simulink model "c2837xD_lcd_display"  (R2021b)
settings: Solver=FixedStepDiscrete  StartTime=0.0  StopTime=Inf  RelTol=1e-3  EnableMultiTasking=on
InitFcn:
  | c2837xD_Display_Param;
values from neighbouring files (symbols this model uses):
  SCI_counter = SCI_ping_buffer_size/SCI_chunk_size    (= 640)    [c2837xD_Display_Param.m]
  SCI_ping_buffer_size = image_height*lines_in_packet    (= 3840)    [c2837xD_Display_Param.m]
  TI_chunk_size = SCI_chunk_size    (= 6)    [c2837xD_Display_Param.m]
  TI_ping_buffer_size = SCI_ping_buffer_size    (= 3840)    [c2837xD_Display_Param.m]
libraries: c280xlib x63, c2837xDlib x63, simulink x41, c2000lib x1, demo_controls x1, dspswit3 x1, idelinklib_common x1
(part 2 of 4)

== system c2837xD_lcd_display/Initialization/GammaCorrection1/Subsystem1 ==
  Cmd : Inport
  Data : Inport  Port=2
  function : TriggerPort  TriggerType=function-call  VariantControl=Variant
  Function-Call Generator : simulink/Ports & Subsystems/Function-Call Generator  sample_time=-1  numberOfIterations=1  DisallowWideOutput=off
  Function-Call Split : FunctionCallSplit  NumOutputPorts=2
  Function-Call Split1 : FunctionCallSplit  NumOutputPorts=2
  Function-Call Split4 : FunctionCallSplit  NumOutputPorts=2
  SendCommand : Subsystem
  SendData : Subsystem
  SetCmd : Subsystem  TreatAsAtomicUnit=on
  SetData : Subsystem  TreatAsAtomicUnit=on
  wires:
  Function-Call Split1/2 -> Function-Call Split4/1
  Function-Call Split/2 -> Function-Call Split1/1
  Data/1 -> SendData/1(Data)
  Function-Call Generator/1 -> Function-Call Split/1
  Function-Call Split/1 -> SetCmd/Trigger
  Function-Call Split4/2 -> SendData/Trigger
  Function-Call Split4/1 -> SetData/Trigger
  Function-Call Split1/1 -> SendCommand/Trigger
  Cmd/1 -> SendCommand/1(cmd)

== system c2837xD_lcd_display/Initialization/GammaCorrection1/Subsystem2 ==
  Cmd : Inport
  Data : Inport  Port=2
  function : TriggerPort  TriggerType=function-call  VariantControl=Variant
  Function-Call Generator : simulink/Ports & Subsystems/Function-Call Generator  sample_time=-1  numberOfIterations=1  DisallowWideOutput=off
  Function-Call Split : FunctionCallSplit  NumOutputPorts=2
  Function-Call Split1 : FunctionCallSplit  NumOutputPorts=2
  Function-Call Split4 : FunctionCallSplit  NumOutputPorts=2
  SendCommand : Subsystem
  SendData : Subsystem
  SetCmd : Subsystem  TreatAsAtomicUnit=on
  SetData : Subsystem  TreatAsAtomicUnit=on
  wires:
  Function-Call Split1/2 -> Function-Call Split4/1
  Function-Call Split/2 -> Function-Call Split1/1
  Data/1 -> SendData/1(Data)
  Function-Call Generator/1 -> Function-Call Split/1
  Function-Call Split/1 -> SetCmd/Trigger
  Function-Call Split4/2 -> SendData/Trigger
  Function-Call Split4/1 -> SetData/Trigger
  Function-Call Split1/1 -> SendCommand/Trigger
  Cmd/1 -> SendCommand/1(cmd)

== system c2837xD_lcd_display/Initialization/GammaCorrection1/Subsystem3 ==
  Cmd : Inport
  Data : Inport  Port=2
  function : TriggerPort  TriggerType=function-call  VariantControl=Variant
  Function-Call Generator : simulink/Ports & Subsystems/Function-Call Generator  sample_time=-1  numberOfIterations=1  DisallowWideOutput=off
  Function-Call Split : FunctionCallSplit  NumOutputPorts=2
  Function-Call Split1 : FunctionCallSplit  NumOutputPorts=2
  Function-Call Split4 : FunctionCallSplit  NumOutputPorts=2
  SendCommand : Subsystem
  SendData : Subsystem
  SetCmd : Subsystem  TreatAsAtomicUnit=on
  SetData : Subsystem  TreatAsAtomicUnit=on
  wires:
  Function-Call Split1/2 -> Function-Call Split4/1
  Function-Call Split/2 -> Function-Call Split1/1
  Data/1 -> SendData/1(Data)
  Function-Call Generator/1 -> Function-Call Split/1
  Function-Call Split/1 -> SetCmd/Trigger
  Function-Call Split4/2 -> SendData/Trigger
  Function-Call Split4/1 -> SetData/Trigger
  Function-Call Split1/1 -> SendCommand/Trigger
  Cmd/1 -> SendCommand/1(cmd)

== system c2837xD_lcd_display/Initialization/GammaCorrection1/Subsystem4 ==
  Cmd : Inport
  Data : Inport  Port=2
  function : TriggerPort  TriggerType=function-call  VariantControl=Variant
  Function-Call Generator : simulink/Ports & Subsystems/Function-Call Generator  sample_time=-1  numberOfIterations=1  DisallowWideOutput=off
  Function-Call Split : FunctionCallSplit  NumOutputPorts=2
  Function-Call Split1 : FunctionCallSplit  NumOutputPorts=2
  Function-Call Split4 : FunctionCallSplit  NumOutputPorts=2
  SendCommand : Subsystem
  SendData : Subsystem
  SetCmd : Subsystem  TreatAsAtomicUnit=on
  SetData : Subsystem  TreatAsAtomicUnit=on
  wires:
  Function-Call Split1/2 -> Function-Call Split4/1
  Function-Call Split/2 -> Function-Call Split1/1
  Data/1 -> SendData/1(Data)
  Function-Call Generator/1 -> Function-Call Split/1
  Function-Call Split/1 -> SetCmd/Trigger
  Function-Call Split4/2 -> SendData/Trigger
  Function-Call Split4/1 -> SetData/Trigger
  Function-Call Split1/1 -> SendCommand/Trigger
  Cmd/1 -> SendCommand/1(cmd)

== system c2837xD_lcd_display/Initialization/InitPwr/Subsystem ==
  Cmd : Inport
  Data : Inport  Port=2
  Function-Call Generator : simulink/Ports & Subsystems/Function-Call Generator  sample_time=-1  numberOfIterations=1  DisallowWideOutput=off
  Function-Call Split : FunctionCallSplit  NumOutputPorts=2
  Function-Call Split1 : FunctionCallSplit  NumOutputPorts=2
  Function-Call Split4 : FunctionCallSplit  NumOutputPorts=2
  SendCommand : Subsystem
  SendData : Subsystem
  SetCmd : Subsystem  TreatAsAtomicUnit=on
  SetData : Subsystem  TreatAsAtomicUnit=on
  wires:
  Function-Call Split1/1 -> SendCommand/Trigger
  Function-Call Generator/1 -> Function-Call Split/1
  Function-Call Split/1 -> SetCmd/Trigger
  Function-Call Split4/2 -> SendData/Trigger
  Function-Call Split4/1 -> SetData/Trigger
  Data/1 -> SendData/1(Data)
  Cmd/1 -> SendCommand/1(cmd)
  Function-Call Split1/2 -> Function-Call Split4/1
  Function-Call Split/2 -> Function-Call Split1/1

== system c2837xD_lcd_display/Initialization/LCDNormal/System Outputs1 ==

== system c2837xD_lcd_display/Initialization/OUTPUT_CTRL_REG/Subsystem ==
  Cmd : Inport
  Data : Inport  Port=2
  Function-Call Generator : simulink/Ports & Subsystems/Function-Call Generator  sample_time=-1  numberOfIterations=1  DisallowWideOutput=off
  Function-Call Split : FunctionCallSplit  NumOutputPorts=2
  Function-Call Split1 : FunctionCallSplit  NumOutputPorts=2
  Function-Call Split4 : FunctionCallSplit  NumOutputPorts=2
  SendCommand : Subsystem
  SendData : Subsystem
  SetCmd : Subsystem  TreatAsAtomicUnit=on
  SetData : Subsystem  TreatAsAtomicUnit=on
  wires:
  Function-Call Split1/1 -> SendCommand/Trigger
  Function-Call Generator/1 -> Function-Call Split/1
  Function-Call Split/1 -> SetCmd/Trigger
  Function-Call Split4/2 -> SendData/Trigger
  Function-Call Split4/1 -> SetData/Trigger
  Data/1 -> SendData/1(Data)
  Cmd/1 -> SendCommand/1(cmd)
  Function-Call Split1/2 -> Function-Call Split4/1
  Function-Call Split/2 -> Function-Call Split1/1

== system c2837xD_lcd_display/Initialization/OscStart/Subsystem ==
  Cmd : Inport
  Data : Inport  Port=2
  Function-Call Generator : simulink/Ports & Subsystems/Function-Call Generator  sample_time=-1  numberOfIterations=1  DisallowWideOutput=off
  Function-Call Split : FunctionCallSplit  NumOutputPorts=2
  Function-Call Split1 : FunctionCallSplit  NumOutputPorts=2
  Function-Call Split4 : FunctionCallSplit  NumOutputPorts=2
  SendCommand : Subsystem
  SendData : Subsystem
  SetCmd : Subsystem  TreatAsAtomicUnit=on
  SetData : Subsystem  TreatAsAtomicUnit=on
  wires:
  Function-Call Split1/1 -> SendCommand/Trigger
  Function-Call Generator/1 -> Function-Call Split/1
  Function-Call Split/1 -> SetCmd/Trigger
  Function-Call Split4/2 -> SendData/Trigger
  Function-Call Split4/1 -> SetData/Trigger
  Data/1 -> SendData/1(Data)
  Cmd/1 -> SendCommand/1(cmd)
  Function-Call Split1/2 -> Function-Call Split4/1
  Function-Call Split/2 -> Function-Call Split1/1

== system c2837xD_lcd_display/Initialization/Reset/COMMAND ==
  function : TriggerPort  TriggerType=function-call  VariantControl=Variant
  System Outputs : Subsystem  mask(System Outputs){ShowInLibBrowser=0}
      mask prompts: ShowInLibBrowser "Simulink:masks:CustCodeMaskParam1_MP"
      settings: CopyFcn=cccopyfcn(gcb)  OpenFcn=ccopenfcn('System Outputs Function')
      mask Help: eval('feval(''rtwprivate'',''rtwhelpview'',''rtw_sys_outputs_block'')');
      mask Display: disp('System\nOutputs');

== system c2837xD_lcd_display/Initialization/Reset/DATA ==
  function : TriggerPort  TriggerType=function-call  VariantControl=Variant
  System Outputs : Subsystem  mask(System Outputs){ShowInLibBrowser=0}
      mask prompts: ShowInLibBrowser "Simulink:masks:CustCodeMaskParam1_MP"
      settings: CopyFcn=cccopyfcn(gcb)  OpenFcn=ccopenfcn('System Outputs Function')
      mask Help: eval('feval(''rtwprivate'',''rtwhelpview'',''rtw_sys_outputs_block'')');
      mask Display: disp('System\nOutputs');

== system c2837xD_lcd_display/Initialization/Reset/DeselectLCD ==
  function : TriggerPort  TriggerType=function-call  VariantControl=Variant
  System Outputs1 : Subsystem  mask(System Outputs){ShowInLibBrowser=0}
      mask prompts: ShowInLibBrowser "Simulink:masks:CustCodeMaskParam1_MP"
      settings: CopyFcn=cccopyfcn(gcb)  OpenFcn=ccopenfcn('System Outputs Function')
      mask Help: eval('feval(''rtwprivate'',''rtwhelpview'',''rtw_sys_outputs_block'')');
      mask Display: disp('System\nOutputs');

== system c2837xD_lcd_display/Initialization/Reset/LCD RESET ==
  function : TriggerPort  TriggerType=function-call  VariantControl=Variant
  System Outputs : Subsystem  mask(System Outputs){ShowInLibBrowser=0}
      mask prompts: ShowInLibBrowser "Simulink:masks:CustCodeMaskParam1_MP"
      settings: CopyFcn=cccopyfcn(gcb)  OpenFcn=ccopenfcn('System Outputs Function')
      mask Help: eval('feval(''rtwprivate'',''rtwhelpview'',''rtw_sys_outputs_block'')');
      mask Display: disp('System\nOutputs');

== system c2837xD_lcd_display/Initialization/Reset/PWM BACKLIGHT ==
  function : TriggerPort  TriggerType=function-call  VariantControl=Variant
  Constant : Constant  SampleTime=-1
  Digital Output : c2837xDlib/Digital Output  GPIO_Number=GPIO0~GPIO7  GPIO_Bit0=on  GPIO_BIT0_Toggle=off  GPIO_Bit1=off  GPIO_BIT1_Toggle=off  GPIO_Bit2=off  GPIO_BIT2_Toggle=off  GPIO_Bit3=off  GPIO_BIT3_Toggle=off  GPIO_Bit4=off  GPIO_BIT4_Toggle=off  GPIO_Bit5=off  GPIO_BIT5_Toggle=off  GPIO_Bit6=off  GPIO_BIT6_Toggle=off  GPIO_Bit7=off  GPIO_BIT7_Toggle=off
      settings: SourceProductBaseCode=TIC2000
  wires:
  Constant/1 -> Digital Output/1

== system c2837xD_lcd_display/Initialization/Reset/SelectLCD ==
  function : TriggerPort  TriggerType=function-call  VariantControl=Variant
  System Outputs1 : Subsystem  mask(System Outputs){ShowInLibBrowser=0}
      mask prompts: ShowInLibBrowser "Simulink:masks:CustCodeMaskParam1_MP"
      settings: CopyFcn=cccopyfcn(gcb)  OpenFcn=ccopenfcn('System Outputs Function')
      mask Help: eval('feval(''rtwprivate'',''rtwhelpview'',''rtw_sys_outputs_block'')');
      mask Display: disp('System\nOutputs');

== system c2837xD_lcd_display/Initialization/SleepMode/Subsystem ==
  Cmd : Inport
  Data : Inport  Port=2
  Function-Call Generator : simulink/Ports & Subsystems/Function-Call Generator  sample_time=-1  numberOfIterations=1  DisallowWideOutput=off
  Function-Call Split : FunctionCallSplit  NumOutputPorts=2
  Function-Call Split1 : FunctionCallSplit  NumOutputPorts=2
  Function-Call Split4 : FunctionCallSplit  NumOutputPorts=2
  SendCommand : Subsystem
  SendData : Subsystem
  SetCmd : Subsystem  TreatAsAtomicUnit=on
  SetData : Subsystem  TreatAsAtomicUnit=on
  wires:
  Function-Call Split1/1 -> SendCommand/Trigger
  Function-Call Generator/1 -> Function-Call Split/1
  Function-Call Split/1 -> SetCmd/Trigger
  Function-Call Split4/2 -> SendData/Trigger
  Function-Call Split4/1 -> SetData/Trigger
  Data/1 -> SendData/1(Data)
  Cmd/1 -> SendCommand/1(cmd)
  Function-Call Split1/2 -> Function-Call Split4/1
  Function-Call Split/2 -> Function-Call Split1/1

== system c2837xD_lcd_display/Initialization/VCOM_OTP_1_REG/Subsystem ==
  Cmd : Inport
  Data : Inport  Port=2
  Function-Call Generator : simulink/Ports & Subsystems/Function-Call Generator  sample_time=-1  numberOfIterations=1  DisallowWideOutput=off
  Function-Call Split : FunctionCallSplit  NumOutputPorts=2
  Function-Call Split1 : FunctionCallSplit  NumOutputPorts=2
  Function-Call Split4 : FunctionCallSplit  NumOutputPorts=2
  SendCommand : Subsystem
  SendData : Subsystem
  SetCmd : Subsystem  TreatAsAtomicUnit=on
  SetData : Subsystem  TreatAsAtomicUnit=on
  wires:
  Function-Call Split1/1 -> SendCommand/Trigger
  Function-Call Generator/1 -> Function-Call Split/1
  Function-Call Split/1 -> SetCmd/Trigger
  Function-Call Split4/2 -> SendData/Trigger
  Function-Call Split4/1 -> SetData/Trigger
  Data/1 -> SendData/1(Data)
  Cmd/1 -> SendCommand/1(cmd)
  Function-Call Split1/2 -> Function-Call Split4/1
  Function-Call Split/2 -> Function-Call Split1/1

== system c2837xD_lcd_display/Initialization/Volt6p1/Subsystem ==
  Cmd : Inport
  Data : Inport  Port=2
  Function-Call Generator : simulink/Ports & Subsystems/Function-Call Generator  sample_time=-1  numberOfIterations=1  DisallowWideOutput=off
  Function-Call Split : FunctionCallSplit  NumOutputPorts=2
  Function-Call Split1 : FunctionCallSplit  NumOutputPorts=2
  Function-Call Split4 : FunctionCallSplit  NumOutputPorts=2
  SendCommand : Subsystem
  SendData : Subsystem
  SetCmd : Subsystem  TreatAsAtomicUnit=on
  SetData : Subsystem  TreatAsAtomicUnit=on
  wires:
  Function-Call Split1/1 -> SendCommand/Trigger
  Function-Call Generator/1 -> Function-Call Split/1
  Function-Call Split/1 -> SetCmd/Trigger
  Function-Call Split4/2 -> SendData/Trigger
  Function-Call Split4/1 -> SetData/Trigger
  Data/1 -> SendData/1(Data)
  Cmd/1 -> SendCommand/1(cmd)
  Function-Call Split1/2 -> Function-Call Split4/1
  Function-Call Split/2 -> Function-Call Split1/1

== system c2837xD_lcd_display/Initialization/Volt6p2/Subsystem ==
  Cmd : Inport
  Data : Inport  Port=2
  function : TriggerPort  TriggerType=function-call  VariantControl=Variant
  Function-Call Generator : simulink/Ports & Subsystems/Function-Call Generator  sample_time=-1  numberOfIterations=1  DisallowWideOutput=off
  Function-Call Split : FunctionCallSplit  NumOutputPorts=2
  Function-Call Split1 : FunctionCallSplit  NumOutputPorts=2
  Function-Call Split4 : FunctionCallSplit  NumOutputPorts=2
  SendCommand : Subsystem
  SendData : Subsystem
  SetCmd : Subsystem  TreatAsAtomicUnit=on
  SetData : Subsystem  TreatAsAtomicUnit=on
  wires:
  Function-Call Split1/2 -> Function-Call Split4/1
  Function-Call Split/2 -> Function-Call Split1/1
  Data/1 -> SendData/1(Data)
  Function-Call Generator/1 -> Function-Call Split/1
  Function-Call Split/1 -> SetCmd/Trigger
  Function-Call Split4/2 -> SendData/Trigger
  Function-Call Split4/1 -> SetData/Trigger
  Function-Call Split1/1 -> SendCommand/Trigger
  Cmd/1 -> SendCommand/1(cmd)

== system c2837xD_lcd_display/Initialization/Volt6p2/Subsystem1 ==
  Cmd : Inport
  Data : Inport  Port=2
  function : TriggerPort  TriggerType=function-call  VariantControl=Variant
  Function-Call Generator : simulink/Ports & Subsystems/Function-Call Generator  sample_time=-1  numberOfIterations=1  DisallowWideOutput=off
  Function-Call Split : FunctionCallSplit  NumOutputPorts=2
  Function-Call Split1 : FunctionCallSplit  NumOutputPorts=2
  Function-Call Split4 : FunctionCallSplit  NumOutputPorts=2
  SendCommand : Subsystem
  SendData : Subsystem
  SetCmd : Subsystem  TreatAsAtomicUnit=on
  SetData : Subsystem  TreatAsAtomicUnit=on
  wires:
  Function-Call Split1/2 -> Function-Call Split4/1
  Function-Call Split/2 -> Function-Call Split1/1
  Data/1 -> SendData/1(Data)
  Function-Call Generator/1 -> Function-Call Split/1
  Function-Call Split/1 -> SetCmd/Trigger
  Function-Call Split4/2 -> SendData/Trigger
  Function-Call Split4/1 -> SetData/Trigger
  Function-Call Split1/1 -> SendCommand/Trigger
  Cmd/1 -> SendCommand/1(cmd)

== system c2837xD_lcd_display/Serial_Interrupt/SCIInterruptEnable/ChangeStatus ==
  IsPong : Inport
  Enable : EnablePort
  ChangePongStatus : Subsystem
  EnableDMAInterrupt : Subsystem
  Function-Call Generator : simulink/Ports & Subsystems/Function-Call Generator  sample_time=-1  numberOfIterations=1  DisallowWideOutput=off
  Function-Call Split : FunctionCallSplit  NumOutputPorts=2
  SPI_PongStatus : Outport  InitialOutput=0  VectorParamsAs1DForOutWhenUnconnected=off
  wires:
  IsPong/1 -> ChangePongStatus/1(IsPong)
  Function-Call Split/2 -> EnableDMAInterrupt/Trigger
  Function-Call Generator/1 -> Function-Call Split/1
  ChangePongStatus/1(SPI_PongStatus) -> SPI_PongStatus/1
  Function-Call Split/1 -> ChangePongStatus/Trigger

== system c2837xD_lcd_display/Serial_Interrupt/SCIInterruptEnable/Counter Logic ==
  DelimiterMatching : Inport
  SCI Counter : Subsystem
  Search for Delimiter : Subsystem
  TogglePingPongStatus : Subsystem  TreatAsAtomicUnit=on
  Delimiter_found : Outport  VectorParamsAs1DForOutWhenUnconnected=off
  CounterValue : Outport  Port=2  VectorParamsAs1DForOutWhenUnconnected=off
  PingPongStatus : Outport  Port=3  VectorParamsAs1DForOutWhenUnconnected=off
  wires:
  TogglePingPongStatus/1(Out1) -> PingPongStatus/1
  Search for Delimiter/1(Delimiter_Found) -> SCI Counter/1(DelimiterFoundStartCounting), Delimiter_found/1
  DelimiterMatching/1 -> Search for Delimiter/1(DelimiterMatching)
  SCI Counter/2(CounterReachedMax) -> TogglePingPongStatus/Enable, Search for Delimiter/2(CounterReachedMax)
  SCI Counter/1(Counter_Value) -> CounterValue/1

== system c2837xD_lcd_display/Serial_Interrupt/SCIInterruptEnable/Detect Ping-Pong Change ==
  In1 : Inport
  Logical Operator : Logic  Operator=XOR  AllPortsSameDT=off  OutDataTypeStr=boolean
  Unit Delay : UnitDelay  SampleTime=-1  HasFrameUpgradeWarning=on
  Out1 : Outport  VectorParamsAs1DForOutWhenUnconnected=off
  wires:
  In1/1 -> Unit Delay/1, Logical Operator/1
  Unit Delay/1 -> Logical Operator/2
  Logical Operator/1 -> Out1/1

== system c2837xD_lcd_display/Serial_Interrupt/SCIInterruptEnable/Is Matching Delimiter ==
  In1 : Inport
  Compare To Delimiter : simulink/Logic and Bit Operations/Compare To Constant  relop===  const=[1 2 3 4 5 6]  OutDataTypeStr=boolean  ZeroCross=off
  Demux : Demux  Outputs=6
  Logical Operator : Logic  Inputs=6  AllPortsSameDT=off  OutDataTypeStr=boolean
  Out1 : Outport  VectorParamsAs1DForOutWhenUnconnected=off
  wires:
  In1/1 -> Compare To Delimiter/1
  Demux/6 -> Logical Operator/6
  Demux/4 -> Logical Operator/4
  Demux/3 -> Logical Operator/3
  Demux/1 -> Logical Operator/1
  Demux/2 -> Logical Operator/2
  Logical Operator/1 -> Out1/1
  Compare To Delimiter/1 -> Demux/1
  Demux/5 -> Logical Operator/5

== system c2837xD_lcd_display/Serial_Interrupt/SCIInterruptEnable/RecordDataIntoPingPongBuffer ==
  AddressCounter : Inport
  IsPong : Inport  Port=2
  Data : Inport  Port=3
  Enable : EnablePort
  Add : Sum  OutDataTypeStr=uint32
  Add1 : Sum  Inputs=+-
  Constant : Constant  OutDataTypeStr=uint16
  Gain : Gain  Gain=TI_chunk_size  ParamDataTypeStr=uint16  OutDataTypeStr=uint16
  Gain1 : Gain  Gain=TI_ping_buffer_size  ParamDataTypeStr=uint16  OutDataTypeStr=uint16
  Memory Copy : idelinklib_common/Memory Copy  copyFrom=Input port  copyFromAddressSource=Specify via dialog  copyFromAddress=hex2dec('00001000')  copyFromSrcCode=myVariableSrc  dataTypeFrom=Inherit from input port  dataDimensionFrom=TI_chunk_size  useOffsetFrom=off  offsetFromSrc=Specify via dialog  offsetFrom=0  strideFrom=1  copyTo=Specified source code symbol  copyToAddressSource=Specify via dialog  copyToAddress=hex2dec('00002000')  copyToSrcCode=Image_Array  dataTypeTo=uint16  useOffsetTo=on  offsetToSrc=Input port  offsetTo=0  strideTo=1  sampleTime=-1  useInitValue=off  initValueSrc=Specify constant value  initValue=1  initValueSrcCode=myInitValueVariable  useAsMask=off  maskOperator=bitwise AND  useTermValue=off  termValue=1  isRealtimeEnabled=off  emitCCBeforeWrite=off  CCBeforeWrite=/* Custom Code Before Write*/  emitCCAfterWrite=off  CCAfterWrite=/* Custom Code After Write*/  useDMACopy=off  enableBlockingMode=off
      settings: SourceProductBaseCode=ME
  Unit Delay : UnitDelay  SampleTime=-1  HasFrameUpgradeWarning=on
  wires:
  Add/1 -> Memory Copy/2
  Gain/1 -> Add/1
  Gain1/1 -> Add/2  "Ping Offset"
  IsPong/1 -> Unit Delay/1
  Unit Delay/1 -> Gain1/1
  AddressCounter/1 -> Add1/1
  Constant/1 -> Add1/2
  Data/1 -> Memory Copy/1
  Add1/1 -> Gain/1

== system c2837xD_lcd_display/Initialization/Analog1/Subsystem/SendCommand ==
  cmd : Inport
  function : TriggerPort  TriggerType=function-call  VariantControl=Variant
  SPI Master Transfer : c280xlib/SPI Master Transfer  SPISelect=SPI_A  ClockPolarity=Rising_edge  ClockPhase=Delay_half_cycle  SPIModule=uint32(0)  Mode=Master  BusSpeed=uint32(1000000)  FirstBitToTransfer=Most significant bit (MSB)  ClockMode=0  BlockFunction=Transfer  EnableRegisterAddress=off  RegisterAddress=0  OutputDataType=int8  OutputDataLength=1  DataBits=8  UseCustomSSPin=Explicit GPIO calls  ActiveLowSSPin=Active low  Pin=124
      settings: SourceProductBaseCode=TIC2000
  Terminator : Terminator
  wires:
  cmd/1 -> SPI Master Transfer/1
  SPI Master Transfer/1 -> Terminator/1

== system c2837xD_lcd_display/Initialization/Analog1/Subsystem/SendData ==
  Data : Inport
  function : TriggerPort  TriggerType=function-call  VariantControl=Variant
  SPI Master Transfer : c280xlib/SPI Master Transfer  SPISelect=SPI_A  ClockPolarity=Rising_edge  ClockPhase=Delay_half_cycle  SPIModule=uint32(0)  Mode=Master  BusSpeed=uint32(1000000)  FirstBitToTransfer=Most significant bit (MSB)  ClockMode=0  BlockFunction=Transfer  EnableRegisterAddress=off  RegisterAddress=0  OutputDataType=int8  OutputDataLength=1  DataBits=8  UseCustomSSPin=Explicit GPIO calls  ActiveLowSSPin=Active low  Pin=124
      settings: SourceProductBaseCode=TIC2000
  Terminator : Terminator
  wires:
  Data/1 -> SPI Master Transfer/1
  SPI Master Transfer/1 -> Terminator/1

== system c2837xD_lcd_display/Initialization/Analog1/Subsystem/SetCmd ==
  function : TriggerPort  TriggerType=function-call  VariantControl=Variant
  Constant : Constant  Value=0  SampleTime=-1
  Digital Output : c2837xDlib/Digital Output  GPIO_Number=GPIO16~GPIO23  GPIO_Bit0=off  GPIO_BIT0_Toggle=off  GPIO_Bit1=off  GPIO_BIT1_Toggle=off  GPIO_Bit2=off  GPIO_BIT2_Toggle=off  GPIO_Bit3=off  GPIO_BIT3_Toggle=off  GPIO_Bit4=off  GPIO_BIT4_Toggle=off  GPIO_Bit5=off  GPIO_BIT5_Toggle=off  GPIO_Bit6=on  GPIO_BIT6_Toggle=off  GPIO_Bit7=off  GPIO_BIT7_Toggle=off
      settings: SourceProductBaseCode=TIC2000
  wires:
  Constant/1 -> Digital Output/1

== system c2837xD_lcd_display/Initialization/Analog1/Subsystem/SetData ==
  function : TriggerPort  TriggerType=function-call  VariantControl=Variant
  Constant1 : Constant  SampleTime=-1
  Digital Output1 : c2837xDlib/Digital Output  GPIO_Number=GPIO16~GPIO23  GPIO_Bit0=off  GPIO_BIT0_Toggle=off  GPIO_Bit1=off  GPIO_BIT1_Toggle=off  GPIO_Bit2=off  GPIO_BIT2_Toggle=off  GPIO_Bit3=off  GPIO_BIT3_Toggle=off  GPIO_Bit4=off  GPIO_BIT4_Toggle=off  GPIO_Bit5=off  GPIO_BIT5_Toggle=off  GPIO_Bit6=on  GPIO_BIT6_Toggle=off  GPIO_Bit7=off  GPIO_BIT7_Toggle=off
      settings: SourceProductBaseCode=TIC2000
  wires:
  Constant1/1 -> Digital Output1/1

== system c2837xD_lcd_display/Initialization/Analog2/Subsystem/SendCommand ==
  cmd : Inport
  function : TriggerPort  TriggerType=function-call  VariantControl=Variant
  SPI Master Transfer : c280xlib/SPI Master Transfer  SPISelect=SPI_A  ClockPolarity=Rising_edge  ClockPhase=Delay_half_cycle  SPIModule=uint32(0)  Mode=Master  BusSpeed=uint32(1000000)  FirstBitToTransfer=Most significant bit (MSB)  ClockMode=0  BlockFunction=Transfer  EnableRegisterAddress=off  RegisterAddress=0  OutputDataType=int8  OutputDataLength=1  DataBits=8  UseCustomSSPin=Explicit GPIO calls  ActiveLowSSPin=Active low  Pin=124
      settings: SourceProductBaseCode=TIC2000
  Terminator : Terminator
  wires:
  cmd/1 -> SPI Master Transfer/1
  SPI Master Transfer/1 -> Terminator/1

== system c2837xD_lcd_display/Initialization/Analog2/Subsystem/SendData ==
  Data : Inport
  function : TriggerPort  TriggerType=function-call  VariantControl=Variant
  SPI Master Transfer : c280xlib/SPI Master Transfer  SPISelect=SPI_A  ClockPolarity=Rising_edge  ClockPhase=Delay_half_cycle  SPIModule=uint32(0)  Mode=Master  BusSpeed=uint32(1000000)  FirstBitToTransfer=Most significant bit (MSB)  ClockMode=0  BlockFunction=Transfer  EnableRegisterAddress=off  RegisterAddress=0  OutputDataType=int8  OutputDataLength=1  DataBits=8  UseCustomSSPin=Explicit GPIO calls  ActiveLowSSPin=Active low  Pin=124
      settings: SourceProductBaseCode=TIC2000
  Terminator : Terminator
  wires:
  Data/1 -> SPI Master Transfer/1
  SPI Master Transfer/1 -> Terminator/1

== system c2837xD_lcd_display/Initialization/Analog2/Subsystem/SetCmd ==
  function : TriggerPort  TriggerType=function-call  VariantControl=Variant
  Constant : Constant  Value=0  SampleTime=-1
  Digital Output : c2837xDlib/Digital Output  GPIO_Number=GPIO16~GPIO23  GPIO_Bit0=off  GPIO_BIT0_Toggle=off  GPIO_Bit1=off  GPIO_BIT1_Toggle=off  GPIO_Bit2=off  GPIO_BIT2_Toggle=off  GPIO_Bit3=off  GPIO_BIT3_Toggle=off  GPIO_Bit4=off  GPIO_BIT4_Toggle=off  GPIO_Bit5=off  GPIO_BIT5_Toggle=off  GPIO_Bit6=on  GPIO_BIT6_Toggle=off  GPIO_Bit7=off  GPIO_BIT7_Toggle=off
      settings: SourceProductBaseCode=TIC2000
  wires:
  Constant/1 -> Digital Output/1

== system c2837xD_lcd_display/Initialization/Analog2/Subsystem/SetData ==
  function : TriggerPort  TriggerType=function-call  VariantControl=Variant
  Constant1 : Constant  SampleTime=-1
  Digital Output1 : c2837xDlib/Digital Output  GPIO_Number=GPIO16~GPIO23  GPIO_Bit0=off  GPIO_BIT0_Toggle=off  GPIO_Bit1=off  GPIO_BIT1_Toggle=off  GPIO_Bit2=off  GPIO_BIT2_Toggle=off  GPIO_Bit3=off  GPIO_BIT3_Toggle=off  GPIO_Bit4=off  GPIO_BIT4_Toggle=off  GPIO_Bit5=off  GPIO_BIT5_Toggle=off  GPIO_Bit6=on  GPIO_BIT6_Toggle=off  GPIO_Bit7=off  GPIO_BIT7_Toggle=off
      settings: SourceProductBaseCode=TIC2000
  wires:
  Constant1/1 -> Digital Output1/1

== system c2837xD_lcd_display/Initialization/AwakeMode/Subsystem/SendCommand ==
  cmd : Inport
  function : TriggerPort  TriggerType=function-call  VariantControl=Variant
  SPI Master Transfer : c280xlib/SPI Master Transfer  SPISelect=SPI_A  ClockPolarity=Rising_edge  ClockPhase=Delay_half_cycle  SPIModule=uint32(0)  Mode=Master  BusSpeed=uint32(1000000)  FirstBitToTransfer=Most significant bit (MSB)  ClockMode=0  BlockFunction=Transfer  EnableRegisterAddress=off  RegisterAddress=0  OutputDataType=int8  OutputDataLength=1  DataBits=8  UseCustomSSPin=Explicit GPIO calls  ActiveLowSSPin=Active low  Pin=124
      settings: SourceProductBaseCode=TIC2000
  Terminator : Terminator
  wires:
  cmd/1 -> SPI Master Transfer/1
  SPI Master Transfer/1 -> Terminator/1

== system c2837xD_lcd_display/Initialization/AwakeMode/Subsystem/SendData ==
  Data : Inport
  function : TriggerPort  TriggerType=function-call  VariantControl=Variant
  SPI Master Transfer : c280xlib/SPI Master Transfer  SPISelect=SPI_A  ClockPolarity=Rising_edge  ClockPhase=Delay_half_cycle  SPIModule=uint32(0)  Mode=Master  BusSpeed=uint32(1000000)  FirstBitToTransfer=Most significant bit (MSB)  ClockMode=0  BlockFunction=Transfer  EnableRegisterAddress=off  RegisterAddress=0  OutputDataType=int8  OutputDataLength=1  DataBits=8  UseCustomSSPin=Explicit GPIO calls  ActiveLowSSPin=Active low  Pin=124
      settings: SourceProductBaseCode=TIC2000
  Terminator : Terminator
  wires:
  Data/1 -> SPI Master Transfer/1
  SPI Master Transfer/1 -> Terminator/1

== system c2837xD_lcd_display/Initialization/AwakeMode/Subsystem/SetCmd ==
  function : TriggerPort  TriggerType=function-call  VariantControl=Variant
  Constant : Constant  Value=0  SampleTime=-1
  Digital Output : c2837xDlib/Digital Output  GPIO_Number=GPIO16~GPIO23  GPIO_Bit0=off  GPIO_BIT0_Toggle=off  GPIO_Bit1=off  GPIO_BIT1_Toggle=off  GPIO_Bit2=off  GPIO_BIT2_Toggle=off  GPIO_Bit3=off  GPIO_BIT3_Toggle=off  GPIO_Bit4=off  GPIO_BIT4_Toggle=off  GPIO_Bit5=off  GPIO_BIT5_Toggle=off  GPIO_Bit6=on  GPIO_BIT6_Toggle=off  GPIO_Bit7=off  GPIO_BIT7_Toggle=off
      settings: SourceProductBaseCode=TIC2000
  wires:
  Constant/1 -> Digital Output/1

== system c2837xD_lcd_display/Initialization/AwakeMode/Subsystem/SetData ==
  function : TriggerPort  TriggerType=function-call  VariantControl=Variant
  Constant1 : Constant  SampleTime=-1
  Digital Output1 : c2837xDlib/Digital Output  GPIO_Number=GPIO16~GPIO23  GPIO_Bit0=off  GPIO_BIT0_Toggle=off  GPIO_Bit1=off  GPIO_BIT1_Toggle=off  GPIO_Bit2=off  GPIO_BIT2_Toggle=off  GPIO_Bit3=off  GPIO_BIT3_Toggle=off  GPIO_Bit4=off  GPIO_BIT4_Toggle=off  GPIO_Bit5=off  GPIO_BIT5_Toggle=off  GPIO_Bit6=on  GPIO_BIT6_Toggle=off  GPIO_Bit7=off  GPIO_BIT7_Toggle=off
      settings: SourceProductBaseCode=TIC2000
  wires:
  Constant1/1 -> Digital Output1/1

== system c2837xD_lcd_display/Initialization/ColorFormat/Subsystem/SendCommand ==
  cmd : Inport
  function : TriggerPort  TriggerType=function-call  VariantControl=Variant
  SPI Master Transfer : c280xlib/SPI Master Transfer  SPISelect=SPI_A  ClockPolarity=Rising_edge  ClockPhase=Delay_half_cycle  SPIModule=uint32(0)  Mode=Master  BusSpeed=uint32(1000000)  FirstBitToTransfer=Most significant bit (MSB)  ClockMode=0  BlockFunction=Transfer  EnableRegisterAddress=off  RegisterAddress=0  OutputDataType=int8  OutputDataLength=1  DataBits=8  UseCustomSSPin=Explicit GPIO calls  ActiveLowSSPin=Active low  Pin=124
      settings: SourceProductBaseCode=TIC2000
  Terminator : Terminator
  wires:
  cmd/1 -> SPI Master Transfer/1
  SPI Master Transfer/1 -> Terminator/1

== system c2837xD_lcd_display/Initialization/ColorFormat/Subsystem/SendData ==
  Data : Inport
  function : TriggerPort  TriggerType=function-call  VariantControl=Variant
  SPI Master Transfer : c280xlib/SPI Master Transfer  SPISelect=SPI_A  ClockPolarity=Rising_edge  ClockPhase=Delay_half_cycle  SPIModule=uint32(0)  Mode=Master  BusSpeed=uint32(1000000)  FirstBitToTransfer=Most significant bit (MSB)  ClockMode=0  BlockFunction=Transfer  EnableRegisterAddress=off  RegisterAddress=0  OutputDataType=int8  OutputDataLength=1  DataBits=8  UseCustomSSPin=Explicit GPIO calls  ActiveLowSSPin=Active low  Pin=124
      settings: SourceProductBaseCode=TIC2000
  Terminator : Terminator
  wires:
  Data/1 -> SPI Master Transfer/1
  SPI Master Transfer/1 -> Terminator/1

== system c2837xD_lcd_display/Initialization/ColorFormat/Subsystem/SetCmd ==
  function : TriggerPort  TriggerType=function-call  VariantControl=Variant
  Constant : Constant  Value=0  SampleTime=-1
  Digital Output : c2837xDlib/Digital Output  GPIO_Number=GPIO16~GPIO23  GPIO_Bit0=off  GPIO_BIT0_Toggle=off  GPIO_Bit1=off  GPIO_BIT1_Toggle=off  GPIO_Bit2=off  GPIO_BIT2_Toggle=off  GPIO_Bit3=off  GPIO_BIT3_Toggle=off  GPIO_Bit4=off  GPIO_BIT4_Toggle=off  GPIO_Bit5=off  GPIO_BIT5_Toggle=off  GPIO_Bit6=on  GPIO_BIT6_Toggle=off  GPIO_Bit7=off  GPIO_BIT7_Toggle=off
      settings: SourceProductBaseCode=TIC2000
  wires:
  Constant/1 -> Digital Output/1

== system c2837xD_lcd_display/Initialization/ColorFormat/Subsystem/SetData ==
  function : TriggerPort  TriggerType=function-call  VariantControl=Variant
  Constant1 : Constant  SampleTime=-1
  Digital Output1 : c2837xDlib/Digital Output  GPIO_Number=GPIO16~GPIO23  GPIO_Bit0=off  GPIO_BIT0_Toggle=off  GPIO_Bit1=off  GPIO_BIT1_Toggle=off  GPIO_Bit2=off  GPIO_BIT2_Toggle=off  GPIO_Bit3=off  GPIO_BIT3_Toggle=off  GPIO_Bit4=off  GPIO_BIT4_Toggle=off  GPIO_Bit5=off  GPIO_BIT5_Toggle=off  GPIO_Bit6=on  GPIO_BIT6_Toggle=off  GPIO_Bit7=off  GPIO_BIT7_Toggle=off
      settings: SourceProductBaseCode=TIC2000
  wires:
  Constant1/1 -> Digital Output1/1

== system c2837xD_lcd_display/Initialization/Data/LCD Data/SendCommand ==
  cmd : Inport
  function : TriggerPort  TriggerType=function-call  VariantControl=Variant
  SPI Master Transfer : c280xlib/SPI Master Transfer  SPISelect=SPI_A  ClockPolarity=Rising_edge  ClockPhase=Delay_half_cycle  SPIModule=uint32(0)  Mode=Master  BusSpeed=uint32(1000000)  FirstBitToTransfer=Most significant bit (MSB)  ClockMode=0  BlockFunction=Transfer  EnableRegisterAddress=off  RegisterAddress=0  OutputDataType=int8  OutputDataLength=1  DataBits=8  UseCustomSSPin=Explicit GPIO calls  ActiveLowSSPin=Active low  Pin=124
      settings: SourceProductBaseCode=TIC2000
  Terminator : Terminator
  wires:
  cmd/1 -> SPI Master Transfer/1
  SPI Master Transfer/1 -> Terminator/1

== system c2837xD_lcd_display/Initialization/Data/LCD Data/SetCmd ==
  function : TriggerPort  TriggerType=function-call  VariantControl=Variant
  Constant : Constant  Value=0  SampleTime=-1
  Digital Output : c2837xDlib/Digital Output  GPIO_Number=GPIO16~GPIO23  GPIO_Bit0=off  GPIO_BIT0_Toggle=off  GPIO_Bit1=off  GPIO_BIT1_Toggle=off  GPIO_Bit2=off  GPIO_BIT2_Toggle=off  GPIO_Bit3=off  GPIO_BIT3_Toggle=off  GPIO_Bit4=off  GPIO_BIT4_Toggle=off  GPIO_Bit5=off  GPIO_BIT5_Toggle=off  GPIO_Bit6=on  GPIO_BIT6_Toggle=off  GPIO_Bit7=off  GPIO_BIT7_Toggle=off
      settings: SourceProductBaseCode=TIC2000
  wires:
  Constant/1 -> Digital Output/1

== system c2837xD_lcd_display/Initialization/Data/LCD Data/SetData ==
  function : TriggerPort  TriggerType=function-call  VariantControl=Variant
  Constant1 : Constant  SampleTime=-1
  Digital Output1 : c2837xDlib/Digital Output  GPIO_Number=GPIO16~GPIO23  GPIO_Bit0=off  GPIO_BIT0_Toggle=off  GPIO_Bit1=off  GPIO_BIT1_Toggle=off  GPIO_Bit2=off  GPIO_BIT2_Toggle=off  GPIO_Bit3=off  GPIO_BIT3_Toggle=off  GPIO_Bit4=off  GPIO_BIT4_Toggle=off  GPIO_Bit5=off  GPIO_BIT5_Toggle=off  GPIO_Bit6=on  GPIO_BIT6_Toggle=off  GPIO_Bit7=off  GPIO_BIT7_Toggle=off
      settings: SourceProductBaseCode=TIC2000
  wires:
  Constant1/1 -> Digital Output1/1

== system c2837xD_lcd_display/Initialization/DataRegister/LCD Data/SendCommand ==
  cmd : Inport
  function : TriggerPort  TriggerType=function-call  VariantControl=Variant
  SPI Master Transfer : c280xlib/SPI Master Transfer  SPISelect=SPI_A  ClockPolarity=Rising_edge  ClockPhase=Delay_half_cycle  SPIModule=uint32(0)  Mode=Master  BusSpeed=uint32(1000000)  FirstBitToTransfer=Most significant bit (MSB)  ClockMode=0  BlockFunction=Transfer  EnableRegisterAddress=off  RegisterAddress=0  OutputDataType=int8  OutputDataLength=1  DataBits=8  UseCustomSSPin=Explicit GPIO calls  ActiveLowSSPin=Active low  Pin=124
      settings: SourceProductBaseCode=TIC2000
  Terminator : Terminator
  wires:
  cmd/1 -> SPI Master Transfer/1
  SPI Master Transfer/1 -> Terminator/1

== system c2837xD_lcd_display/Initialization/DataRegister/LCD Data/SendData ==
  Data : Inport
  function : TriggerPort  TriggerType=function-call  VariantControl=Variant
  SendData : Subsystem
  wires:
  Data/1 -> SendData/1(Data1)

== system c2837xD_lcd_display/Initialization/DataRegister/LCD Data/SetCmd ==
  function : TriggerPort  TriggerType=function-call  VariantControl=Variant
  Constant : Constant  Value=0  SampleTime=-1
  Digital Output : c2837xDlib/Digital Output  GPIO_Number=GPIO16~GPIO23  GPIO_Bit0=off  GPIO_BIT0_Toggle=off  GPIO_Bit1=off  GPIO_BIT1_Toggle=off  GPIO_Bit2=off  GPIO_BIT2_Toggle=off  GPIO_Bit3=off  GPIO_BIT3_Toggle=off  GPIO_Bit4=off  GPIO_BIT4_Toggle=off  GPIO_Bit5=off  GPIO_BIT5_Toggle=off  GPIO_Bit6=on  GPIO_BIT6_Toggle=off  GPIO_Bit7=off  GPIO_BIT7_Toggle=off
      settings: SourceProductBaseCode=TIC2000
  wires:
  Constant/1 -> Digital Output/1

== system c2837xD_lcd_display/Initialization/DataRegister/LCD Data/SetData ==
  function : TriggerPort  TriggerType=function-call  VariantControl=Variant
  Constant1 : Constant  SampleTime=-1
  Digital Output1 : c2837xDlib/Digital Output  GPIO_Number=GPIO16~GPIO23  GPIO_Bit0=off  GPIO_BIT0_Toggle=off  GPIO_Bit1=off  GPIO_BIT1_Toggle=off  GPIO_Bit2=off  GPIO_BIT2_Toggle=off  GPIO_Bit3=off  GPIO_BIT3_Toggle=off  GPIO_Bit4=off  GPIO_BIT4_Toggle=off  GPIO_Bit5=off  GPIO_BIT5_Toggle=off  GPIO_Bit6=on  GPIO_BIT6_Toggle=off  GPIO_Bit7=off  GPIO_BIT7_Toggle=off
      settings: SourceProductBaseCode=TIC2000
  wires:
  Constant1/1 -> Digital Output1/1

== system c2837xD_lcd_display/Initialization/DispEnable/Subsystem/SendCommand ==
  cmd : Inport
  function : TriggerPort  TriggerType=function-call  VariantControl=Variant
  SPI Master Transfer : c280xlib/SPI Master Transfer  SPISelect=SPI_A  ClockPolarity=Rising_edge  ClockPhase=Delay_half_cycle  SPIModule=uint32(0)  Mode=Master  BusSpeed=uint32(1000000)  FirstBitToTransfer=Most significant bit (MSB)  ClockMode=0  BlockFunction=Transfer  EnableRegisterAddress=off  RegisterAddress=0  OutputDataType=int8  OutputDataLength=1  DataBits=8  UseCustomSSPin=Explicit GPIO calls  ActiveLowSSPin=Active low  Pin=124
      settings: SourceProductBaseCode=TIC2000
  Terminator : Terminator
  wires:
  cmd/1 -> SPI Master Transfer/1
  SPI Master Transfer/1 -> Terminator/1

== system c2837xD_lcd_display/Initialization/DispEnable/Subsystem/SendData ==
  Data : Inport
  function : TriggerPort  TriggerType=function-call  VariantControl=Variant
  SPI Master Transfer : c280xlib/SPI Master Transfer  SPISelect=SPI_A  ClockPolarity=Rising_edge  ClockPhase=Delay_half_cycle  SPIModule=uint32(0)  Mode=Master  BusSpeed=uint32(1000000)  FirstBitToTransfer=Most significant bit (MSB)  ClockMode=0  BlockFunction=Transfer  EnableRegisterAddress=off  RegisterAddress=0  OutputDataType=int8  OutputDataLength=1  DataBits=8  UseCustomSSPin=Explicit GPIO calls  ActiveLowSSPin=Active low  Pin=124
      settings: SourceProductBaseCode=TIC2000
  Terminator : Terminator
  wires:
  Data/1 -> SPI Master Transfer/1
  SPI Master Transfer/1 -> Terminator/1

== system c2837xD_lcd_display/Initialization/DispEnable/Subsystem/SetCmd ==
  function : TriggerPort  TriggerType=function-call  VariantControl=Variant
  Constant : Constant  Value=0  SampleTime=-1
  Digital Output : c2837xDlib/Digital Output  GPIO_Number=GPIO16~GPIO23  GPIO_Bit0=off  GPIO_BIT0_Toggle=off  GPIO_Bit1=off  GPIO_BIT1_Toggle=off  GPIO_Bit2=off  GPIO_BIT2_Toggle=off  GPIO_Bit3=off  GPIO_BIT3_Toggle=off  GPIO_Bit4=off  GPIO_BIT4_Toggle=off  GPIO_Bit5=off  GPIO_BIT5_Toggle=off  GPIO_Bit6=on  GPIO_BIT6_Toggle=off  GPIO_Bit7=off  GPIO_BIT7_Toggle=off
      settings: SourceProductBaseCode=TIC2000
  wires:
  Constant/1 -> Digital Output/1

== system c2837xD_lcd_display/Initialization/DispEnable/Subsystem/SetData ==
  function : TriggerPort  TriggerType=function-call  VariantControl=Variant
  Constant1 : Constant  SampleTime=-1
  Digital Output1 : c2837xDlib/Digital Output  GPIO_Number=GPIO16~GPIO23  GPIO_Bit0=off  GPIO_BIT0_Toggle=off  GPIO_Bit1=off  GPIO_BIT1_Toggle=off  GPIO_Bit2=off  GPIO_BIT2_Toggle=off  GPIO_Bit3=off  GPIO_BIT3_Toggle=off  GPIO_Bit4=off  GPIO_BIT4_Toggle=off  GPIO_Bit5=off  GPIO_BIT5_Toggle=off  GPIO_Bit6=on  GPIO_BIT6_Toggle=off  GPIO_Bit7=off  GPIO_BIT7_Toggle=off
      settings: SourceProductBaseCode=TIC2000
  wires:
  Constant1/1 -> Digital Output1/1

== system c2837xD_lcd_display/Initialization/DispOrient/Subsystem/SendCommand ==
  cmd : Inport
  function : TriggerPort  TriggerType=function-call  VariantControl=Variant
  SPI Master Transfer : c280xlib/SPI Master Transfer  SPISelect=SPI_A  ClockPolarity=Rising_edge  ClockPhase=Delay_half_cycle  SPIModule=uint32(0)  Mode=Master  BusSpeed=uint32(1000000)  FirstBitToTransfer=Most significant bit (MSB)  ClockMode=0  BlockFunction=Transfer  EnableRegisterAddress=off  RegisterAddress=0  OutputDataType=int8  OutputDataLength=1  DataBits=8  UseCustomSSPin=Explicit GPIO calls  ActiveLowSSPin=Active low  Pin=124
      settings: SourceProductBaseCode=TIC2000
  Terminator : Terminator
  wires:
  cmd/1 -> SPI Master Transfer/1
  SPI Master Transfer/1 -> Terminator/1

== system c2837xD_lcd_display/Initialization/DispOrient/Subsystem/SendData ==
  Data : Inport
  function : TriggerPort  TriggerType=function-call  VariantControl=Variant
  SPI Master Transfer : c280xlib/SPI Master Transfer  SPISelect=SPI_A  ClockPolarity=Rising_edge  ClockPhase=Delay_half_cycle  SPIModule=uint32(0)  Mode=Master  BusSpeed=uint32(1000000)  FirstBitToTransfer=Most significant bit (MSB)  ClockMode=0  BlockFunction=Transfer  EnableRegisterAddress=off  RegisterAddress=0  OutputDataType=int8  OutputDataLength=1  DataBits=8  UseCustomSSPin=Explicit GPIO calls  ActiveLowSSPin=Active low  Pin=124
      settings: SourceProductBaseCode=TIC2000
  Terminator : Terminator
  wires:
  Data/1 -> SPI Master Transfer/1
  SPI Master Transfer/1 -> Terminator/1

== system c2837xD_lcd_display/Initialization/DispOrient/Subsystem/SetCmd ==
  function : TriggerPort  TriggerType=function-call  VariantControl=Variant
  Constant : Constant  Value=0  SampleTime=-1
  Digital Output : c2837xDlib/Digital Output  GPIO_Number=GPIO16~GPIO23  GPIO_Bit0=off  GPIO_BIT0_Toggle=off  GPIO_Bit1=off  GPIO_BIT1_Toggle=off  GPIO_Bit2=off  GPIO_BIT2_Toggle=off  GPIO_Bit3=off  GPIO_BIT3_Toggle=off  GPIO_Bit4=off  GPIO_BIT4_Toggle=off  GPIO_Bit5=off  GPIO_BIT5_Toggle=off  GPIO_Bit6=on  GPIO_BIT6_Toggle=off  GPIO_Bit7=off  GPIO_BIT7_Toggle=off
      settings: SourceProductBaseCode=TIC2000
  wires:
  Constant/1 -> Digital Output/1

== system c2837xD_lcd_display/Initialization/DispOrient/Subsystem/SetData ==
  function : TriggerPort  TriggerType=function-call  VariantControl=Variant
  Constant1 : Constant  SampleTime=-1
  Digital Output1 : c2837xDlib/Digital Output  GPIO_Number=GPIO16~GPIO23  GPIO_Bit0=off  GPIO_BIT0_Toggle=off  GPIO_Bit1=off  GPIO_BIT1_Toggle=off  GPIO_Bit2=off  GPIO_BIT2_Toggle=off  GPIO_Bit3=off  GPIO_BIT3_Toggle=off  GPIO_Bit4=off  GPIO_BIT4_Toggle=off  GPIO_Bit5=off  GPIO_BIT5_Toggle=off  GPIO_Bit6=on  GPIO_BIT6_Toggle=off  GPIO_Bit7=off  GPIO_BIT7_Toggle=off
      settings: SourceProductBaseCode=TIC2000
  wires:
  Constant1/1 -> Digital Output1/1

== system c2837xD_lcd_display/Initialization/GRAMWindow/Subsystem/SendCommand ==
  cmd : Inport
  function : TriggerPort  TriggerType=function-call  VariantControl=Variant
  SPI Master Transfer : c280xlib/SPI Master Transfer  SPISelect=SPI_A  ClockPolarity=Rising_edge  ClockPhase=Delay_half_cycle  SPIModule=uint32(0)  Mode=Master  BusSpeed=uint32(1000000)  FirstBitToTransfer=Most significant bit (MSB)  ClockMode=0  BlockFunction=Transfer  EnableRegisterAddress=off  RegisterAddress=0  OutputDataType=int8  OutputDataLength=1  DataBits=8  UseCustomSSPin=Explicit GPIO calls  ActiveLowSSPin=Active low  Pin=124
      settings: SourceProductBaseCode=TIC2000
  Terminator : Terminator
  wires:
  cmd/1 -> SPI Master Transfer/1
  SPI Master Transfer/1 -> Terminator/1

== system c2837xD_lcd_display/Initialization/GRAMWindow/Subsystem/SendData ==
  Data : Inport
  function : TriggerPort  TriggerType=function-call  VariantControl=Variant
  SPI Master Transfer : c280xlib/SPI Master Transfer  SPISelect=SPI_A  ClockPolarity=Rising_edge  ClockPhase=Delay_half_cycle  SPIModule=uint32(0)  Mode=Master  BusSpeed=uint32(1000000)  FirstBitToTransfer=Most significant bit (MSB)  ClockMode=0  BlockFunction=Transfer  EnableRegisterAddress=off  RegisterAddress=0  OutputDataType=int8  OutputDataLength=1  DataBits=8  UseCustomSSPin=Explicit GPIO calls  ActiveLowSSPin=Active low  Pin=124
      settings: SourceProductBaseCode=TIC2000
  Terminator : Terminator
  wires:
  Data/1 -> SPI Master Transfer/1
  SPI Master Transfer/1 -> Terminator/1

== system c2837xD_lcd_display/Initialization/GRAMWindow/Subsystem/SetCmd ==
  function : TriggerPort  TriggerType=function-call  VariantControl=Variant
  Constant : Constant  Value=0  SampleTime=-1
  Digital Output : c2837xDlib/Digital Output  GPIO_Number=GPIO16~GPIO23  GPIO_Bit0=off  GPIO_BIT0_Toggle=off  GPIO_Bit1=off  GPIO_BIT1_Toggle=off  GPIO_Bit2=off  GPIO_BIT2_Toggle=off  GPIO_Bit3=off  GPIO_BIT3_Toggle=off  GPIO_Bit4=off  GPIO_BIT4_Toggle=off  GPIO_Bit5=off  GPIO_BIT5_Toggle=off  GPIO_Bit6=on  GPIO_BIT6_Toggle=off  GPIO_Bit7=off  GPIO_BIT7_Toggle=off
      settings: SourceProductBaseCode=TIC2000
  wires:
  Constant/1 -> Digital Output/1

== system c2837xD_lcd_display/Initialization/GRAMWindow/Subsystem/SetData ==
  function : TriggerPort  TriggerType=function-call  VariantControl=Variant
  Constant1 : Constant  SampleTime=-1
  Digital Output1 : c2837xDlib/Digital Output  GPIO_Number=GPIO16~GPIO23  GPIO_Bit0=off  GPIO_BIT0_Toggle=off  GPIO_Bit1=off  GPIO_BIT1_Toggle=off  GPIO_Bit2=off  GPIO_BIT2_Toggle=off  GPIO_Bit3=off  GPIO_BIT3_Toggle=off  GPIO_Bit4=off  GPIO_BIT4_Toggle=off  GPIO_Bit5=off  GPIO_BIT5_Toggle=off  GPIO_Bit6=on  GPIO_BIT6_Toggle=off  GPIO_Bit7=off  GPIO_BIT7_Toggle=off
      settings: SourceProductBaseCode=TIC2000
  wires:
  Constant1/1 -> Digital Output1/1

== system c2837xD_lcd_display/Initialization/GRAMWindow/Subsystem1/SendCommand ==
  cmd : Inport
  function : TriggerPort  TriggerType=function-call  VariantControl=Variant
  SPI Master Transfer : c280xlib/SPI Master Transfer  SPISelect=SPI_A  ClockPolarity=Rising_edge  ClockPhase=Delay_half_cycle  SPIModule=uint32(0)  Mode=Master  BusSpeed=uint32(1000000)  FirstBitToTransfer=Most significant bit (MSB)  ClockMode=0  BlockFunction=Transfer  EnableRegisterAddress=off  RegisterAddress=0  OutputDataType=int8  OutputDataLength=1  DataBits=8  UseCustomSSPin=Explicit GPIO calls  ActiveLowSSPin=Active low  Pin=124
      settings: SourceProductBaseCode=TIC2000
  Terminator : Terminator
  wires:
  cmd/1 -> SPI Master Transfer/1
  SPI Master Transfer/1 -> Terminator/1

== system c2837xD_lcd_display/Initialization/GRAMWindow/Subsystem1/SendData ==
  Data : Inport
  function : TriggerPort  TriggerType=function-call  VariantControl=Variant
  SPI Master Transfer : c280xlib/SPI Master Transfer  SPISelect=SPI_A  ClockPolarity=Rising_edge  ClockPhase=Delay_half_cycle  SPIModule=uint32(0)  Mode=Master  BusSpeed=uint32(1000000)  FirstBitToTransfer=Most significant bit (MSB)  ClockMode=0  BlockFunction=Transfer  EnableRegisterAddress=off  RegisterAddress=0  OutputDataType=int8  OutputDataLength=1  DataBits=8  UseCustomSSPin=Explicit GPIO calls  ActiveLowSSPin=Active low  Pin=124
      settings: SourceProductBaseCode=TIC2000
  Terminator : Terminator
  wires:
  Data/1 -> SPI Master Transfer/1
  SPI Master Transfer/1 -> Terminator/1

== system c2837xD_lcd_display/Initialization/GRAMWindow/Subsystem1/SetCmd ==
  function : TriggerPort  TriggerType=function-call  VariantControl=Variant
  Constant : Constant  Value=0  SampleTime=-1
  Digital Output : c2837xDlib/Digital Output  GPIO_Number=GPIO16~GPIO23  GPIO_Bit0=off  GPIO_BIT0_Toggle=off  GPIO_Bit1=off  GPIO_BIT1_Toggle=off  GPIO_Bit2=off  GPIO_BIT2_Toggle=off  GPIO_Bit3=off  GPIO_BIT3_Toggle=off  GPIO_Bit4=off  GPIO_BIT4_Toggle=off  GPIO_Bit5=off  GPIO_BIT5_Toggle=off  GPIO_Bit6=on  GPIO_BIT6_Toggle=off  GPIO_Bit7=off  GPIO_BIT7_Toggle=off
      settings: SourceProductBaseCode=TIC2000
  wires:
  Constant/1 -> Digital Output/1

== system c2837xD_lcd_display/Initialization/GRAMWindow/Subsystem1/SetData ==
  function : TriggerPort  TriggerType=function-call  VariantControl=Variant
  Constant1 : Constant  SampleTime=-1
  Digital Output1 : c2837xDlib/Digital Output  GPIO_Number=GPIO16~GPIO23  GPIO_Bit0=off  GPIO_BIT0_Toggle=off  GPIO_Bit1=off  GPIO_BIT1_Toggle=off  GPIO_Bit2=off  GPIO_BIT2_Toggle=off  GPIO_Bit3=off  GPIO_BIT3_Toggle=off  GPIO_Bit4=off  GPIO_BIT4_Toggle=off  GPIO_Bit5=off  GPIO_BIT5_Toggle=off  GPIO_Bit6=on  GPIO_BIT6_Toggle=off  GPIO_Bit7=off  GPIO_BIT7_Toggle=off
      settings: SourceProductBaseCode=TIC2000
  wires:
  Constant1/1 -> Digital Output1/1

== system c2837xD_lcd_display/Initialization/GRAMWindow/Subsystem2/SendCommand ==
  cmd : Inport
  function : TriggerPort  TriggerType=function-call  VariantControl=Variant
  SPI Master Transfer : c280xlib/SPI Master Transfer  SPISelect=SPI_A  ClockPolarity=Rising_edge  ClockPhase=Delay_half_cycle  SPIModule=uint32(0)  Mode=Master  BusSpeed=uint32(1000000)  FirstBitToTransfer=Most significant bit (MSB)  ClockMode=0  BlockFunction=Transfer  EnableRegisterAddress=off  RegisterAddress=0  OutputDataType=int8  OutputDataLength=1  DataBits=8  UseCustomSSPin=Explicit GPIO calls  ActiveLowSSPin=Active low  Pin=124
      settings: SourceProductBaseCode=TIC2000
  Terminator : Terminator
  wires:
  cmd/1 -> SPI Master Transfer/1
  SPI Master Transfer/1 -> Terminator/1

== system c2837xD_lcd_display/Initialization/GRAMWindow/Subsystem2/SendData ==
  Data : Inport
  function : TriggerPort  TriggerType=function-call  VariantControl=Variant
  SPI Master Transfer : c280xlib/SPI Master Transfer  SPISelect=SPI_A  ClockPolarity=Rising_edge  ClockPhase=Delay_half_cycle  SPIModule=uint32(0)  Mode=Master  BusSpeed=uint32(1000000)  FirstBitToTransfer=Most significant bit (MSB)  ClockMode=0  BlockFunction=Transfer  EnableRegisterAddress=off  RegisterAddress=0  OutputDataType=int8  OutputDataLength=1  DataBits=8  UseCustomSSPin=Explicit GPIO calls  ActiveLowSSPin=Active low  Pin=124
      settings: SourceProductBaseCode=TIC2000
  Terminator : Terminator
  wires:
  Data/1 -> SPI Master Transfer/1
  SPI Master Transfer/1 -> Terminator/1

== system c2837xD_lcd_display/Initialization/GRAMWindow/Subsystem2/SetCmd ==
  function : TriggerPort  TriggerType=function-call  VariantControl=Variant
  Constant : Constant  Value=0  SampleTime=-1
  Digital Output : c2837xDlib/Digital Output  GPIO_Number=GPIO16~GPIO23  GPIO_Bit0=off  GPIO_BIT0_Toggle=off  GPIO_Bit1=off  GPIO_BIT1_Toggle=off  GPIO_Bit2=off  GPIO_BIT2_Toggle=off  GPIO_Bit3=off  GPIO_BIT3_Toggle=off  GPIO_Bit4=off  GPIO_BIT4_Toggle=off  GPIO_Bit5=off  GPIO_BIT5_Toggle=off  GPIO_Bit6=on  GPIO_BIT6_Toggle=off  GPIO_Bit7=off  GPIO_BIT7_Toggle=off
      settings: SourceProductBaseCode=TIC2000
  wires:
  Constant/1 -> Digital Output/1
